simulink subsystem "StudentTemplate_MTMTMAD006_M2_FINAL"  (R2025a)
settings: Solver=VariableStepAuto  StartTime=0.0  StopTime=10.0  RelTol=1e-3
libraries: simulink x10, slpidlib x10, eeGeneralControl x3, dspstat3 x3, cstblocks x1
(part 3 of 3)

== stateflow chart StudentTemplate_MTMTMAD006_M2_FINAL/draft2_Maze_exploration2 ==
  settings: updateMethod=CONTINUOUS  sampleTime=0.005
  state Left_turn1
    entry:
    theta = Z_theta;
    Z_angle = Z_angle +pi/2;
    during:
    LW = -1;
    RW = 1;
    exit:
    turn_indicator = 1
  state Go_straight
    during:
    LW = 1;
    RW = 1;
  state left_turn_setup
    entry:
    start_dist = dist_trav;
    end_dist = start_dist + 0.145;
  state Go_straight1
    entry:
    turn_indicator = 0;
    during:
    LW = 1;
    RW = 1;
  state set_Z_angle
    entry:
    Z_angle = 0;
  state Start
    entry:
    LW = 0;
    RW =0;
    turn_indicator = 0;
  state Full_rotation
    entry:
    theta = Z_theta;
    Z_angle = Z_angle - pi;
    during:
    LW = 1;
    RW =-1;
    exit:
    turn_indicator = 1;
  state Left_turn
    entry:
    theta = Z_theta;
    Z_angle = Z_angle + pi/2;
    during:
    LW = -1;
    RW = 1;
    exit:
    turn_indicator = 1;
  state Left_turn2
    entry:
    theta = Z_theta;
    Z_angle = Z_angle +pi/2;
    during:
    LW = -1;
    RW = 1;
    exit:
    turn_indicator = 1;
  state left_turn_setup1
    entry:
    start_dist = dist_trav;
    end_dist = start_dist + 0.145;
  state right_turn
    entry:
    theta =Z_theta;
    Z_angle = Z_angle - pi/2;
    during:
    LW = 1;
    RW =-1;
    exit:
    turn_indicator = 1;
  left_turn_setup -> Left_turn1 [order 2] : [dist_trav >= end_dist  || TOF_F == 1 && TOF_L == 0 ]
  Go_straight -> left_turn_setup [order 2] : [TOF_F ==0 && TOF_L ==0]
  Start -> Go_straight [order 4] : [TOF_L == 1 && TOF_F == 0 || TOF_R == 1 && TOF_F ==0]
  Go_straight -> (junction 107) [order 1] : [TOF_F ==1  ]
  Left_turn1 -> Go_straight1 : [Z_theta >= Z_angle]
  left_turn_setup -> (junction 103) [order 1] : [TOF_L ==1 ]
  (default) -> set_Z_angle
  (junction 103) -> (junction 107)
  Go_straight1 -> (junction 103) [order 1] : [TOF_F ==1  ]
  left_turn_setup1 -> (junction 103) [order 1] : [TOF_L ==1 ]
  (junction 107) -> Start
  Full_rotation -> (junction 103) : [Z_theta <= Z_angle && TOF_F == 0 ]
  set_Z_angle -> Start
  Go_straight1 -> left_turn_setup1 [order 2] : [TOF_F ==0 && TOF_L ==0]
  Start -> Full_rotation [order 1] : [TOF_L == 1 && TOF_R == 1 && TOF_F ==1]
  Start -> Left_turn [order 2] : [TOF_L ==0 && TOF_F ==1]
  Left_turn2 -> Start : [Z_theta >= Z_angle]
  Left_turn -> Start : [Z_theta >= Z_angle]
  right_turn -> Start : [Z_theta <= Z_angle]
  Start -> right_turn [order 3] : [TOF_R ==0 && TOF_F ==1]
  left_turn_setup1 -> Left_turn2 [order 2] : [dist_trav >= end_dist || TOF_F == 1 && TOF_L == 0  ]
  data: TOF_L input; TOF_R input; LW output; RW output; dist_trav input; start_dist local; TOF_F input; end_dist local; Z_theta input; turn_indicator output; theta local; Z_angle output
